simulink library "flowAtNodeDepths_cl"  (R2018b)
settings: Solver=VariableStepAuto  StartTime=0.0  StopTime=10.0  RelTol=1e-3
settings Model: Creator=James Reed  LastModifiedBy=James Reed

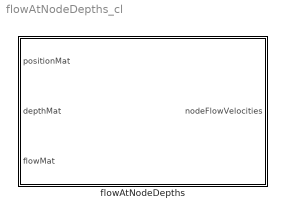
== system flowAtNodeDepths_cl ==
  "flowAtNodeDepths " : Subsystem

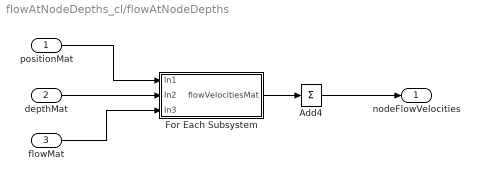
== system flowAtNodeDepths_cl/flowAtNodeDepths  ==
  "positionMat " : Inport
  depthMat : Inport  Port=2
  flowMat : Inport  Port=3
  Add4 : Sum  Inputs=1  CollapseMode=Specified dimension  CollapseDim=2
  For Each Subsystem : Subsystem  TreatAsAtomicUnit=on
  nodeFlowVelocities : Outport
  wires:
  flowMat/1 -> For Each Subsystem/3(In3)
  Add4/1 -> nodeFlowVelocities/1
  depthMat/1 -> For Each Subsystem/2(In2)
  For Each Subsystem/1("flowVelocitiesMat ") -> Add4/1
  "positionMat "/1 -> For Each Subsystem/1(In1)

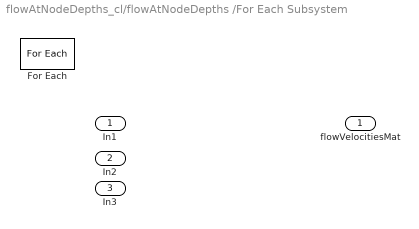
== system flowAtNodeDepths_cl/flowAtNodeDepths /For Each Subsystem ==
  In1 : Inport  Partition=on  PartitionDimension=1  PartitionWidth=1  PartitionOffset=0
  In2 : Inport  Port=2  Partition=on  PartitionDimension=1  PartitionWidth=1  PartitionOffset=0
  In3 : Inport  Port=3  Partition=on  PartitionDimension=1  PartitionWidth=1  PartitionOffset=0
  For Each : ForEach  DisableCoverage=on  IndexMode=One-based
  "flowVelocitiesMat " : Outport  ConcatenationDimension=1
